simulink model "PIntkVUs_VD"  (R2016b)
settings: configuration reference "CodeGenConfigSet" (kept outside this file)
values from neighbouring files (symbols this model uses):
  Air_dpGradLimPIntkVUs_C = Calibration.Parameter    [init_PIntkVUs_VD.m]
  Air_facPT1T1SigPIntkVUs_C = Calibration.Parameter    [init_PIntkVUs_VD.m]
  Air_pTransStgPIntkVUsDfl_C = Calibration.Parameter    [init_PIntkVUs_VD.m]
  Air_RmpSlpPIntkVUsNeg_C = Calibration.Parameter    [init_PIntkVUs_VD.m]
  Air_RmpSlpPIntkVUsPos_C = Calibration.Parameter    [init_PIntkVUs_VD.m]
  SigTst_pPIntkVUs_C = Calibration.Parameter    [init_PIntkVUs_VD.m]
  SigTst_swtPIntkVUs_C = Calibration.Parameter    [init_PIntkVUs_VD.m]
undefined symbols (not defined in the file or in its folder): CEngDst_switch_conv, PIntkVUs_VD_DT, Switch_conv
libraries: CXLib x6
settings Model: Creator=GaberXu  LastModifiedBy=GaberXu
settings ConfigSetRef: SourceLocation=Base Workspace

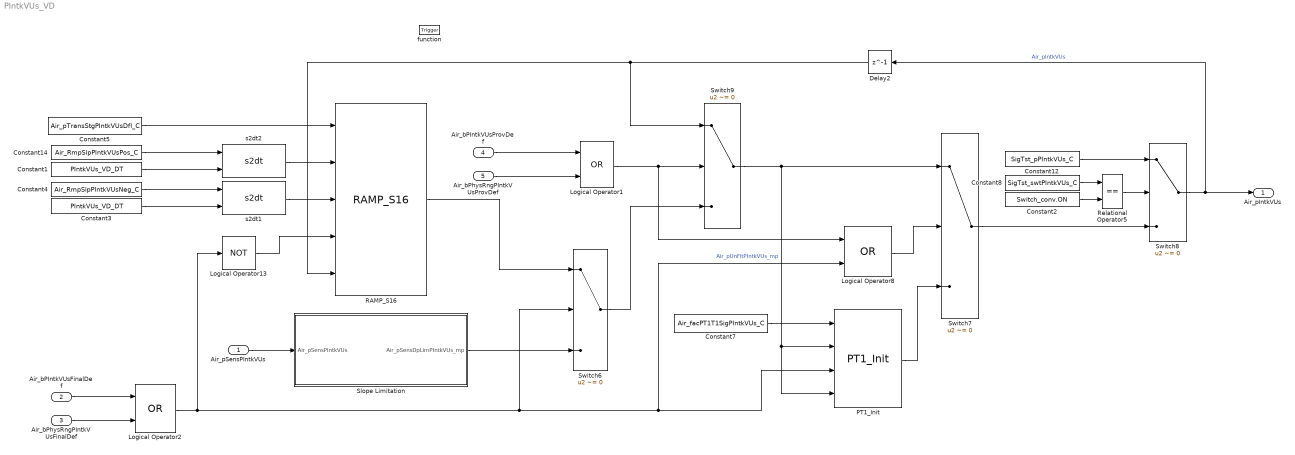
== system PIntkVUs_VD ==
  Air_pSensPIntkVUs : Inport  Tag=kPa  Description=Sensed manifold absolute pressure  OutMin=0  OutMax=1200  OutDataTypeStr=AirPressure_kPa
  Air_bPIntkVUsFinalDef : Inport  Description=Final defect of the raw air pressure upstream of the intake valve  Port=2  OutMin=0  OutMax=1  OutDataTypeStr=boolean
  Air_bPhysRngPIntkVUsFinalDef : Inport  Description=Final defect of the physical air pressure upstream of the intake valve  Port=3  OutMin=0  OutMax=1  OutDataTypeStr=boolean
  Air_bPIntkVUsProvDef : Inport  Description=Provisional defect of the raw air pressure upstream of the intake valve  Port=4  OutMin=0  OutMax=1  OutDataTypeStr=boolean
  Air_bPhysRngPIntkVUsProvDef : Inport  Description=Provisional defect of the physical air pressure upstream of the intake valve  Port=5  OutMin=0  OutMax=1  OutDataTypeStr=boolean
  function : TriggerPort  TriggerType=function-call  VariantControl=Variant
  Constant1 : Constant  Value=PIntkVUs_VD_DT
  Constant12 : Constant  RequirementInfo={'other' 'CEngDsT_requirements.doc' '@Simulink_requirement_item_6' 'true' '手动冷却水温值' '' } %GIDa_7aba2ff8_3549_4659_a362_760b5a80f2a7  Value=SigTst_pPIntkVUs_C  SampleTime=-1
  Constant14 : Constant  RequirementInfo={'other' 'CEngDsT_requirements.doc' '@Simulink_requirement_item_8' 'true' '冷却水温故障时斜坡至默认值' '' } %GIDa_918f64f1_4a30_4fc3_83e0_3f25f5ca48b5  Value=Air_RmpSlpPIntkVUsPos_C  SampleTime=-1
  Constant2 : Constant  RequirementInfo={'other' 'APP_requirements.doc' '@Simulink_requirement_item_25' 'true' '手动开关' '' } %GIDa_37ec2c05_5bcb_4764_95f9_4a96450e4b04  Value=Switch_conv.ON  OutDataTypeStr=Inherit: Inherit via back propagation
  Constant3 : Constant  Value=PIntkVUs_VD_DT
  Constant4 : Constant  RequirementInfo={'other' 'CEngDsT_requirements.doc' '@Simulink_requirement_item_8' 'true' '冷却水温故障时斜坡至默认值' '' } %GIDa_8aca41e5_ce5b_47ca_a422_aa2e6fd71d9c  Value=Air_RmpSlpPIntkVUsNeg_C  SampleTime=-1
  Constant5 : Constant  RequirementInfo={'other' 'CEngDsT_requirements.doc' '@Simulink_requirement_item_8' 'true' '冷却水温故障时斜坡至默认值' '' } %GIDa_b2f26015_8c53_41ff_8759_7afaab8069ff  Value=Air_pTransStgPIntkVUsDfl_C  SampleTime=-1
  Constant7 : Constant  Value=Air_facPT1T1SigPIntkVUs_C  SampleTime=-1
  Constant8 : Constant  RequirementInfo={'other' 'CEngDsT_requirements.doc' '@Simulink_requirement_item_6' 'true' '手动冷却水温值' '' } %GIDa_d3914eca_6432_43cf_a4fa_20e66f944c76  Value=SigTst_swtPIntkVUs_C  SampleTime=-1
  Delay2 : Delay  DialogController=Simulink.DDGSource  DelayLength=1  InitialCondition=0
  Logical Operator1 : Logic  Operator=OR  OutDataTypeStr=boolean
  Logical Operator13 : Logic  Operator=NOT  AllPortsSameDT=off  OutDataTypeStr=boolean
  Logical Operator2 : Logic  Operator=OR  OutDataTypeStr=boolean
  Logical Operator8 : Logic  Operator=OR  OutDataTypeStr=boolean
  PT1_Init : CXLib/PT1_Init
  RAMP_S16 : CXLib/RAMP_S16  RequirementInfo={'other' 'CEngDsT_requirements.doc' '@Simulink_requirement_item_8' 'true' '冷却水温故障时斜坡至默认值' '' } %GIDa_a801b524_22e9_425d_913e_8ae68e19156f
  Relational Operator5 : RelationalOperator  Operator===  OutDataTypeStr=boolean  RndMeth=Simplest  InputSameDT=on
  Slope Limitation : Subsystem
  Switch6 : Switch  Criteria=u2 ~= 0  InputSameDT=on
  Switch7 : Switch  RequirementInfo={'other' 'CEngDsT_requirements.doc' '@Simulink_requirement_item_5' 'true' '冷却水温滤波去抖动' '' } %GIDa_109ffbe6_4ce9_40b4_b730_3904e7ec5ebf  Criteria=u2 ~= 0  InputSameDT=on
  Switch8 : Switch  RequirementInfo={'other' 'CEngDsT_requirements.doc' '@Simulink_requirement_item_6' 'true' '手动冷却水温值' '' } %GIDa_3c6bc85a_2caa_4b8b_ab2f_c6722522d191  Criteria=u2 ~= 0  Threshold=CEngDst_switch_conv.OFF  InputSameDT=on
  Switch9 : Switch  Criteria=u2 ~= 0  InputSameDT=on
  s2dt1 : CXLib/s2dt
  s2dt2 : CXLib/s2dt
  Air_pIntkVUs : Outport  Tag=kPa  Description=Intake valve upstream pressure  OutMin=0  OutMax=1200  OutDataTypeStr=AirPressure_kPa
  wires:
  Air_pSensPIntkVUs/1 -> Slope Limitation/1(Air_pSensPIntkVUs)
  Delay2/1 -> RAMP_S16/5, Switch9/1
  Switch9/1 -> Switch7/1, PT1_Init/4, PT1_Init/2  "Air_pUnFltPIntkVUs_mp"
  Switch6/1 -> Switch9/3
  Logical Operator8/1 -> Switch7/2
  Switch7/1 -> Switch8/3
  Switch8/1 -> Air_pIntkVUs/1, Delay2/1  "Air_pIntkVUs"
  Constant5/1 -> RAMP_S16/1
  Logical Operator2/1 -> PT1_Init/3, Logical Operator8/2, Switch6/2, Logical Operator13/1
  Logical Operator13/1 -> RAMP_S16/4
  Constant12/1 -> Switch8/1
  s2dt2/1 -> RAMP_S16/2
  s2dt1/1 -> RAMP_S16/3
  Constant7/1 -> PT1_Init/1
  RAMP_S16/1 -> Switch6/1
  PT1_Init/1 -> Switch7/3
  Relational Operator5/1 -> Switch8/2
  Constant8/1 -> Relational Operator5/1
  Constant2/1 -> Relational Operator5/2
  Slope Limitation/1(Air_pSensDpLimPIntkVUs_mp) -> Switch6/3
  Constant14/1 -> s2dt2/1
  Constant1/1 -> s2dt2/2
  Constant4/1 -> s2dt1/1
  Constant3/1 -> s2dt1/2
  Air_bPhysRngPIntkVUsFinalDef/1 -> Logical Operator2/2
  Air_bPIntkVUsFinalDef/1 -> Logical Operator2/1
  Air_bPIntkVUsProvDef/1 -> Logical Operator1/1
  Air_bPhysRngPIntkVUsProvDef/1 -> Logical Operator1/2
  Logical Operator1/1 -> Logical Operator8/1, Switch9/2

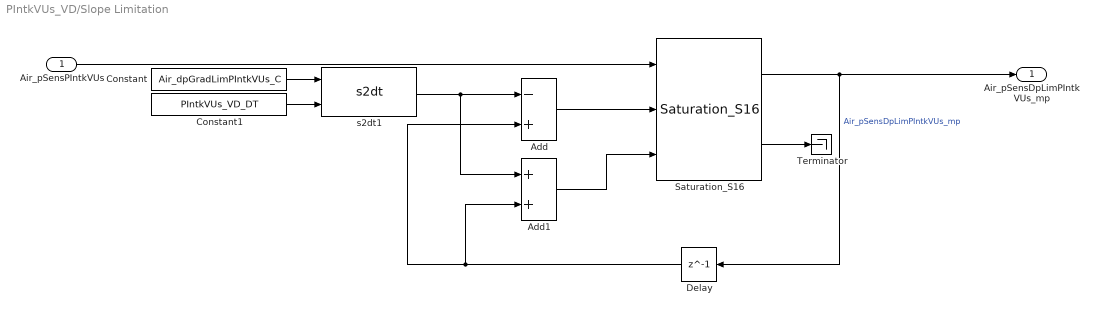
== system PIntkVUs_VD/Slope Limitation ==
  Air_pSensPIntkVUs : Inport
  Add : Sum  Inputs=-+  InputSameDT=on
  Add1 : Sum  InputSameDT=on
  Constant : Constant  Value=Air_dpGradLimPIntkVUs_C
  Constant1 : Constant  Value=PIntkVUs_VD_DT
  Delay : Delay  DelayLength=1  InitialCondition=0
  Saturation_S16 : CXLib/Saturation_S16
  Terminator : Terminator
  s2dt1 : CXLib/s2dt
  Air_pSensDpLimPIntkVUs_mp : Outport
  wires:
  Saturation_S16/2 -> Terminator/1
  Add1/1 -> Saturation_S16/3
  Add/1 -> Saturation_S16/2
  Delay/1 -> Add/2, Add1/2
  Saturation_S16/1 -> Delay/1, Air_pSensDpLimPIntkVUs_mp/1  "Air_pSensDpLimPIntkVUs_mp"
  Air_pSensPIntkVUs/1 -> Saturation_S16/1
  s2dt1/1 -> Add1/1, Add/1
  Constant/1 -> s2dt1/1
  Constant1/1 -> s2dt1/2
